simulink model "ringBufferPitch"  (R2022a)
settings: Solver=VariableStepAuto  StartTime=0.0  StopTime=simParams.stopTime  RelTol=1e-3
PostLoadFcn:
  | postLoadCallback
InitFcn:
  | initCallback
StopFcn:
  | stopCallback
undefined symbols (not defined in the file): buffer_bit_num, buffer_size, frac_Nbits, modelParams
libraries: hdlsllib x5, embmathops x3, dspsrcs4 x1
CloseFcn:
  | closeCallback
settings Model: Creator=ronne  LastModifiedBy=Connor Watz
settings DataIOCC: ReturnWorkspaceOutputs=off
settings OptimizationCC: BlockReduction=off  ConditionallyExecuteInputs=off  DefaultParameterBehavior=Inlined
settings DebuggingCC: AlgebraicLoopMsg=error  UnconnectedInputMsg=warning  UnconnectedOutputMsg=warning  UnconnectedLineMsg=warning
settings HardwareCC: ProdBitPerPointer=32  ProdBitPerSizeT=32  ProdBitPerPtrDiffT=32  ProdLargestAtomicFloat=None  ProdIntDivRoundTo=Undefined  ProdEndianess=Unspecified  ProdWordSize=32  ProdHWDeviceType=ASIC/FPGA->ASIC/FPGA  TargetBitPerPointer=64  TargetBitPerSizeT=64  TargetBitPerPtrDiffT=64  TargetLongLongMode=on  TargetIntDivRoundTo=Zero  TargetEndianess=LittleEndian  TargetWordSize=64  TargetHWDeviceType=Custom Processor->MATLAB Host Computer  ProdEqTarget=off
settings RTWCC: DLArmComputeVersion=19.05

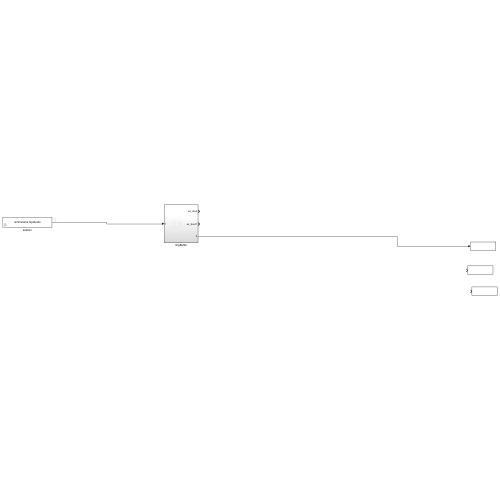
[thumbnail: Simulink's stored preview of the top-level diagram]
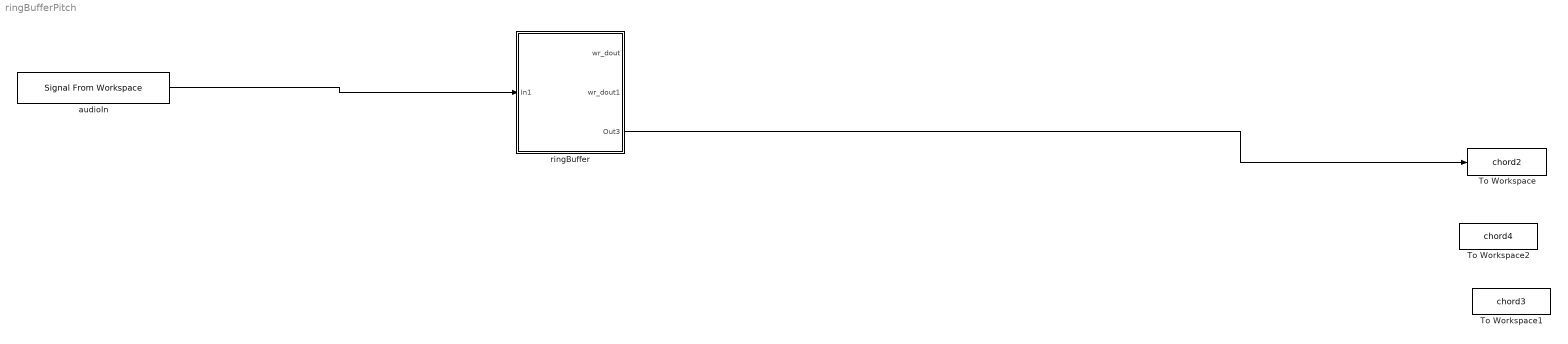
== system ringBufferPitch ==
  To Workspace : ToWorkspace  VariableName=chord2  SaveFormat=Timeseries  SampleTime=-1
  To Workspace1 : ToWorkspace  VariableName=chord3  SaveFormat=Timeseries  SampleTime=-1
  To Workspace2 : ToWorkspace  VariableName=chord4  SaveFormat=Timeseries  SampleTime=-1
  audioIn : dspsrcs4/Signal From Workspace  X=simParams.fxptAudio  Ts=modelParams.audio.samplePeriod  nsamps=1  OutputAfterFinalValue=Setting to zero  ignoreOrWarnInputAndFrameLengths=off  OutputFrames=off
  ringBuffer : Subsystem
  wires:
  audioIn/1 -> ringBuffer/1(In1)
  ringBuffer/3(Out3) -> To Workspace/1

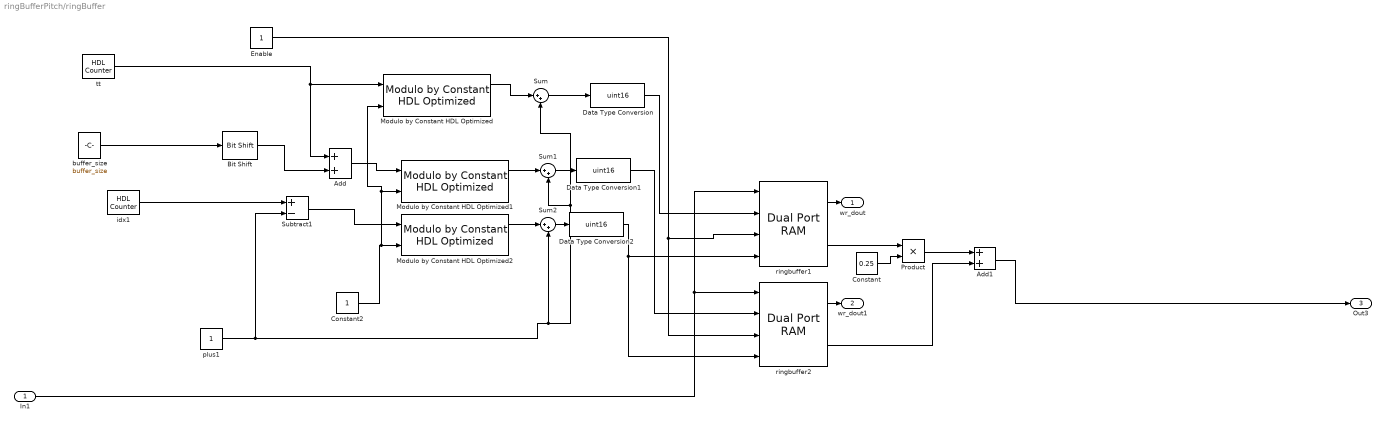
== system ringBufferPitch/ringBuffer ==
  In1 : Inport
  Add : Sum
  Add1 : Sum  OutDataTypeStr=Inherit: Inherit via back propagation
  Bit Shift : hdlsllib/Logic and Bit Operations/Bit Shift  mode=Shift Right Logical  N=1
  Constant : Constant  Value=0.25  OutDataTypeStr=Inherit: Inherit via back propagation
  Constant2 : Constant  OutDataTypeStr=boolean  SampleTime=-1
  Data Type Conversion : DataTypeConversion  OutDataTypeStr=uint16  SaturateOnIntegerOverflow=off  RndMeth=Floor
  Data Type Conversion1 : DataTypeConversion  OutDataTypeStr=uint16  SaturateOnIntegerOverflow=off  RndMeth=Floor
  Data Type Conversion2 : DataTypeConversion  OutDataTypeStr=uint16  SaturateOnIntegerOverflow=off  RndMeth=Floor
  Enable : Constant  OutDataTypeStr=boolean
  Modulo by Constant HDL Optimized : embmathops/Modulo by Constant HDL Optimized  Denominator=1024  SimulateUsing=Code generation
      settings: SourceProductBaseCode=SL
  Modulo by Constant HDL Optimized1 : embmathops/Modulo by Constant HDL Optimized  Denominator=1024  SimulateUsing=Code generation
      settings: SourceProductBaseCode=SL
  Modulo by Constant HDL Optimized2 : embmathops/Modulo by Constant HDL Optimized  Denominator=1024  SimulateUsing=Code generation
      settings: SourceProductBaseCode=SL
  Product : Product  OutDataTypeStr=Inherit: Inherit via back propagation
  Subtract1 : Sum  Inputs=+-  OutDataTypeStr=Inherit: Inherit via back propagation
  Sum : Sum  Inputs=|++  OutDataTypeStr=Inherit: Same as first input
  Sum1 : Sum  Inputs=|++  OutDataTypeStr=Inherit: Same as first input
  Sum2 : Sum  Inputs=|++  OutDataTypeStr=Inherit: Same as first input
  buffer_size : Constant  Value=buffer_size  SampleTime=modelParams.audio.samplePeriod
  idx1 : hdlsllib/Sources/HDL Counter  CountType=Free running  CountInit=delta1  CountStep=delta1  CountMax=25  CountFromType=Initial value  CountFrom=delta1  CountResetPort=off  CountLoadPort=off  CountEnbPort=off  CountDirPort=off  CountHitOutputPort=off  CountDataType=Unsigned  CountWordLen=buffer_bit_num + frac_Nbits  CountFracLen=frac_Nbits  CountSampTime=modelParams.audio.samplePeriod
  plus1 : Constant  OutDataTypeStr=Inherit: Inherit via back propagation  SampleTime=-1
  ringbuffer1 : hdlsllib/HDL RAMs/Dual Port RAM  ram_size=16
      settings: SourceProductBaseCode=SL
  ringbuffer2 : hdlsllib/HDL RAMs/Dual Port RAM  ram_size=16
      settings: SourceProductBaseCode=SL
  tt : hdlsllib/Sources/HDL Counter  CountType=Free running  CountInit=1  CountStep=1  CountMax=25  CountFromType=Initial value  CountFrom=1  CountResetPort=off  CountLoadPort=off  CountEnbPort=off  CountDirPort=off  CountHitOutputPort=off  CountDataType=Unsigned  CountWordLen=10  CountFracLen=0  CountSampTime=modelParams.audio.samplePeriod
  wr_dout : Outport
  wr_dout1 : Outport  Port=2
  Out3 : Outport  Port=3
  wires:
  Bit Shift/1 -> Add/2
  Add/1 -> Modulo by Constant HDL Optimized1/1
  tt/1 -> Modulo by Constant HDL Optimized/1, Add/1
  Subtract1/1 -> Modulo by Constant HDL Optimized2/1
  ringbuffer2/2 -> Add1/2
  Sum/1 -> Data Type Conversion/1
  Enable/1 -> ringbuffer2/3, ringbuffer1/3
  Sum1/1 -> Data Type Conversion1/1
  Modulo by Constant HDL Optimized1/1 -> Sum1/1
  In1/1 -> ringbuffer2/1, ringbuffer1/1
  Constant/1 -> Product/2
  Modulo by Constant HDL Optimized2/1 -> Sum2/1
  buffer_size/1 -> Bit Shift/1
  Add1/1 -> Out3/1
  ringbuffer1/2 -> Product/1
  Sum2/1 -> Data Type Conversion2/1
  idx1/1 -> Subtract1/1
  Modulo by Constant HDL Optimized/1 -> Sum/1
  Product/1 -> Add1/1
  ringbuffer2/1 -> wr_dout1/1
  ringbuffer1/1 -> wr_dout/1
  plus1/1 -> Sum/2, Sum1/2, Sum2/2, Subtract1/2
  Constant2/1 -> Modulo by Constant HDL Optimized/2, Modulo by Constant HDL Optimized1/2, Modulo by Constant HDL Optimized2/2
  Data Type Conversion/1 -> ringbuffer1/2
  Data Type Conversion1/1 -> ringbuffer2/2
  Data Type Conversion2/1 -> ringbuffer2/4, ringbuffer1/4
